simulink model "roll_control"  (R2020b)
settings: Solver=VariableStepAuto  StartTime=0.0  StopTime=3.45  FixedStep=0.001  RelTol=1e-5  AbsTol=1e-6
PostLoadFcn:
  | path = fileparts(which(bdroot))
  | cd(path)
  | masscgI = xlsread('mass,cg,I','mass,cg,I');
  | ThrustTable = xlsread('F15_Thrust','Sheet1');
  | u = xlsread('../../scp_new_problem/src/u.csv','u');
InitFcn:
  | HeightAboveSeaLevel = 5.4419142084;
  | 
  | GustStart = 1;
  | GustLength = [120, 130, 80];
  | GuestAmplitude = [ 2.5, -2.5,  1];
  | 
  | ShearSpeed = 4;
  | ShearDirection = 75;
  | 
  | Croll = 0.001 * (rand - 0.5);
  | Cyaw = 0.05 * (rand - 0.5);
  | Cside = 0.001 * (rand - 0.5);
  | 
  | GustStart = 2 * rand;
  | GustLength = [100 + 50 * (rand - 0.5), 100 + 50 * (rand - 0.5), 100 + 50 * (rand - 0.5)];
  | GuestAmplitude = [ 5 * (rand - 0.5), 5 * (rand - 0.5),  5 * (rand - 0.5)];
  | 
  | ShearSpeed = 5 * rand;
  | ShearDirection = 360 * rand;
  | 
  | HeightAboveSeaLevel = rand * 1000;
values from neighbouring files (symbols this model uses):
  cg = temp(4)    [NonlinearStateEstimationForActuatorDelay.m]
  D = zeros(size(B))    [RocketOutputFunction.m]    (also in StateSpaceController.m; TimeDelayCompensationElevator.m = [0; 0])
  F = eye(6)    [MEKFAttitudeOnly.m]
  I = reshape(x(1:9), [3 3])    [AdaptiveLQR.m]    (also in MEKF.m = diag([0.08 0.08 0.002]); MEKFAttitudeOnly.m = diag([0.08 0.08 0.002]); MEKF_old.m = diag([0.08 0.08 0.002]); NonlinearStateEstimationForActuatorDelay.m = diag([Ixx, Ixx, Izz]))
  K = 1.1    [DATCOMvsOR.m]    (also in Forces_and_Moments_Calculator.m; MEKF.m = (P * H.') / (H * P * H.' + V); MEKFAttitudeOnly.m = P2 * H' * inv(S); MEKF_old.m = (P * H.') / (H * P * H.' + V))
  mass = 1.0565    [ImpactVelocityNotParallelMatlab.m]    (also in NonlinearStateEstimationForActuatorDelay.m = temp(1); OneDLanding.m; RunImpactVelocityParforCompiled.m; StateSpaceController.m = 1.0616753546)
  q = x(13:16)    [AdaptiveLQR.m]    (also in MEKF.m = nominal_state(4:7); MEKFAttitudeOnly.m = [1 0 0 0]; MEKF_old.m = nominal_state(4:7); NonlinearStateEstimationForActuatorDelay.m = x(4:7))
  r = [0; 0; -(rocket_length - Average_cg)]    [StateSpaceController.m]    (also in TimeDelayCompensationElevator.m = [0;0]; Tracker.m)
  s = linspace(0, 100, nums)    [ImpactVelocityFunction.m]    (also in ImpactVelocityNotParallelMatlab.m = 1:5:500; ParallelImpactVelocity.m = .1:.01:500; ParralelRun.m = linspace(5,7, nums); RunImpactVelocityParforCompiled.m = 1:0.1:500)
  whentoignite = [s(row); v(col)]    [SecondPartLandingAlgorithm.m]
undefined symbols (not defined in the file or in its folder): Angle, Axis, deg, e0_0, e1_0, e2_0, e3_0, Earth, Kri, Light, magnitude, MIL, rad, WGS84
libraries: aerolibutil x7, vrlib x6, shared6dof x6, aerolibconvert2 x5, simulink x4, sharedtransform x4, aerolibwind2 x3, pid_lib x3, robotcorelib x2, sharedutil x2, aerolibasang x2, aerolibatmos2 x1
(part 1 of 3)
settings Model: ExtModeTrigDuration=100  OrderedModelArguments=off  Creator=rag  LastModifiedBy=rag
settings SolverCC: MaxConsecutiveZCs=10000  ZeroCrossAlgorithm=Adaptive  MinimalZcImpactIntegration=on
settings DataIOCC: Decimation=1000000  SaveOutput=off  DSMLogging=off  ReturnWorkspaceOutputs=off  StateSaveName=tmp_raccel_xout  SignalLoggingName=tmp_raccel_logsout  Refine=2
settings OptimizationCC: EfficientMapNaN2IntZero=off  SimCompilerOptimization=on
settings DebuggingCC: ReadBeforeWriteMsg=DisableAll  WriteAfterWriteMsg=DisableAll  WriteAfterReadMsg=DisableAll  AlgebraicLoopMsg=error
settings HardwareCC: ProdHWDeviceType=AMD->x86-64 (Windows64)  TargetBitPerPointer=64  TargetBitPerSizeT=64  TargetBitPerPtrDiffT=64  TargetLongLongMode=on  TargetIntDivRoundTo=Zero  TargetEndianess=LittleEndian  TargetWordSize=64  TargetHWDeviceType=MATLAB Host  ProdEqTarget=off
settings ModelReferenceCC: UpdateModelReferenceTargets=IfOutOfDate
settings SFSimCC: SFSimEcho=off  CustomCodeUndefinedFunction=UseInterfaceOnly
settings RTWCC: SystemTargetFile=raccel.tlc  TemplateMakefile=raccel_default_tmf  RTWVerbose=off  RTWUseSimCustomCode=on
settings CodeAppCC: GenerateComments=off  MaxIdLength=128  MangleLength=10
settings RaccelTargetCC: ENABLE_SLEXEC_SSBRIDGE=1  RTWCAPIParams=on  RTWCAPIRootIO=off
settings ConfigComp: CovScope=ReferencedModels

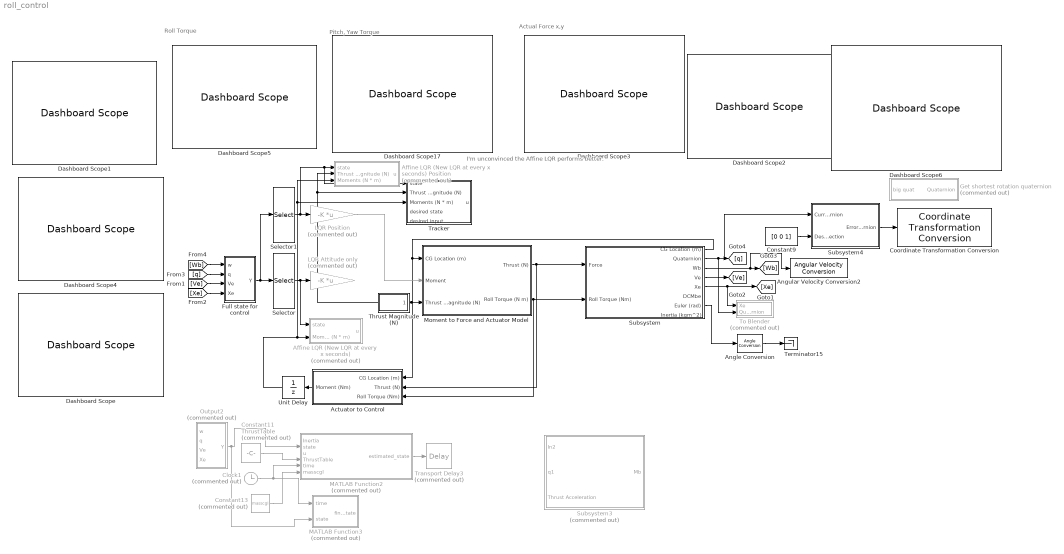
== system roll_control ==
  note: I'm unconvinced the Affine LQR performs better.
  note: Actual Force x,y
  note: Pitch, Yaw Torque
  note: Roll Torque
  Actuator to Control : Subsystem
  Affine LQR (New LQR at every x seconds) : Subsystem  Commented=on
  Affine LQR (New LQR at every x seconds) Position : Subsystem  Commented=on
  Angle Conversion : aerolibconvert2/Angle Conversion  IU=rad  OU=deg
  Angular Velocity Conversion2 : aerolibconvert2/Angular Velocity Conversion  IU=rad/s  OU=deg/s
  Clock1 : Clock  Commented=on
  Constant11 : Constant  Commented=on  Value=ThrustTable
  Constant13 : Constant  Commented=on  Value=masscgI
  Constant9 : Constant  Value=[0 0 1]
  Coordinate Transformation Conversion : robotcorelib/Coordinate Transformation Conversion  InputRepresentation=Quaternion  InputEulerSequence=ZYX  ShowTrVecInputPort=on  OutputRepresentation=Axis-Angle  OutputEulerSequence=ZYX  ShowTrVecOutputPort=on  SimulateUsing=Code generation
      settings: SourceProductBaseCode=NV,RO,RR,UV
  Dashboard Scope{,1..4,6} (6 alike) : DashboardScope
  Dashboard Scope17 : DashboardScope  TimeSpan=3.4500000000000002
  Dashboard Scope5 : DashboardScope  TimeSpan=3.4500000000000002
  Full state for control : Subsystem
  Get shortest rotation quaternion : Subsystem  Commented=on
  LQR Attitude only : Gain  Commented=on  Gain=-K  Multiplication=Matrix(K*u) (u vector)
  LQR Position : Gain  Commented=on  Gain=-K  Multiplication=Matrix(K*u) (u vector)
  MATLAB Function2 : MATLAB Function  Commented=on  TreatAsAtomicUnit=on
  MATLAB Function3 : MATLAB Function  Commented=on  TreatAsAtomicUnit=on
  Moment to Force and Actuator Model : Subsystem
  Output2 : Subsystem  Commented=on
  Selector : Selector  InputPortWidth=13  IndexOptions=Index vector (dialog)  Indices=[1:9]  OutputSizes=1
  Selector1 : Selector  InputPortWidth=13  IndexOptions=Index vector (dialog)  Indices=[1:6, 10:13]  OutputSizes=1
  Subsystem : Subsystem
  Subsystem3 : Subsystem  Commented=on
  Subsystem4 : Subsystem
  Terminator15 : Terminator
  Thrust Magnitude (N) : Subsystem
  To Blender : Subsystem  Commented=on
  Tracker : Subsystem
  Transport Delay3 : TransportDelay  Commented=on  DelayTime=0.5  TransDelayFeedthrough=on
  Unit Delay : UnitDelay  SampleTime=-1  HasFrameUpgradeWarning=on
  wires:
  Constant9/1 -> Subsystem4/2(Desired Direction)
  Constant11/1 -> MATLAB Function2/4(ThrustTable)
  Clock1/1 -> MATLAB Function2/5(time), MATLAB Function3/1(time)
  Output2/1(Y) -> MATLAB Function3/2(state), MATLAB Function2/2(state)
  Constant13/1 -> MATLAB Function2/6(masscgI)
  Subsystem/1(CG Location (m)) -> Actuator to Control/1(CG Location (m)), Moment to Force and Actuator Model/1(CG Location (m))
  Moment to Force and Actuator Model/1(Thrust (N)) -> Subsystem/1(Force), Actuator to Control/2(Thrust (N))
  Moment to Force and Actuator Model/2(Roll Torque (N m)) -> Subsystem/2(Roll Torque (Nm)), Actuator to Control/3(Roll Torque (Nm))
  MATLAB Function2/1(estimated_state) -> Transport Delay3/1
  Thrust Magnitude (N)/1(Thrust Magnitude (N)) -> Moment to Force and Actuator Model/3(Thrust Magnitude (N)), Affine LQR (New LQR at every x seconds) Position/2(Thrust Magnitude (N)), Tracker/2(Thrust Magnitude (N))
  Subsystem4/1(Error Quaternion) -> Coordinate Transformation Conversion/1
  Subsystem/5(Xe) -> To Blender/1(Xe), [Xe]
  [Xe] -> Full state for control/4(Xe)
  Subsystem/3(Wb) -> Angular Velocity Conversion2/1, [Wb]
  Subsystem/4(Ve) -> [Ve]
  Subsystem/2(Quaternion) -> To Blender/2(Quaternion), Subsystem4/1(Current Quaternion), [q]
  [Ve] -> Full state for control/3(Ve)
  [Wb] -> Full state for control/1(w)
  [q] -> Full state for control/2(q)
  Full state for control/1(Y) -> Selector1/1, Selector/1
  Selector/1 -> Affine LQR (New LQR at every x seconds)/1(state), LQR Attitude only/1
  Angle Conversion/1 -> Terminator15/1
  Subsystem/7(Euler (rad)) -> Angle Conversion/1
  Selector1/1 -> Tracker/1(state), Affine LQR (New LQR at every x seconds) Position/1(state), LQR Position/1
  Actuator to Control/1(Moment (Nm)) -> Unit Delay/1
  Unit Delay/1 -> Affine LQR (New LQR at every x seconds) Position/3(Moments (N * m)), Tracker/3(Moments (N * m)), Affine LQR (New LQR at every x seconds)/2(Moments (N * m))
  LQR Position/1 -> Moment to Force and Actuator Model/2(Moment)

== system roll_control/Actuator to Control ==
  CG Location (m) : Inport
  Thrust (N) : Inport  Port=2
  Roll Torque (Nm) : Inport  Port=3
  1 : Constant  Value=[0 0]
  Actuator to moment : Subsystem
  Mux : Mux  Inputs=2
  Sum : Sum  Inputs=|++
  Moment (Nm) : Outport
  wires:
  Actuator to moment/1(Thrust moment) -> Sum/1
  1/1 -> Mux/1
  Mux/1 -> Sum/2
  Roll Torque (Nm)/1 -> Mux/2
  Sum/1 -> Moment (Nm)/1
  CG Location (m)/1 -> Actuator to moment/1(CG Location (m))
  Thrust (N)/1 -> Actuator to moment/2(Thrust (N))

== system roll_control/Affine LQR (New LQR at every x seconds) ==
  state : Inport
  Moments (N * m) : Inport  Port=2
  Clock : Clock
  MATLAB Function1 : MATLAB Function  TreatAsAtomicUnit=on
  Matrix Multiply : Product  Multiplication=Matrix(*)
  Sum : Sum  Inputs=|--
  u : Outport
  wires:
  Clock/1 -> MATLAB Function1/3(time)
  state/1 -> Matrix Multiply/2, MATLAB Function1/1(state)
  Sum/1 -> u/1
  Matrix Multiply/1 -> Sum/1
  MATLAB Function1/2(k_0_out) -> Sum/2
  MATLAB Function1/1(K_x_out) -> Matrix Multiply/1
  Moments (N * m)/1 -> MATLAB Function1/2(u)

== system roll_control/Affine LQR (New LQR at every x seconds) Position ==
  state : Inport
  Thrust Magnitude (N) : Inport  Port=2
  Moments (N * m) : Inport  Port=3
  Clock : Clock
  MATLAB Function1 : MATLAB Function  TreatAsAtomicUnit=on
  Matrix Multiply : Product  Multiplication=Matrix(*)
  Sum : Sum  Inputs=|--
  u : Outport
  wires:
  Clock/1 -> MATLAB Function1/3(time)
  state/1 -> MATLAB Function1/1(state), Matrix Multiply/2
  Sum/1 -> u/1
  Matrix Multiply/1 -> Sum/1
  MATLAB Function1/2(k_0_out) -> Sum/2
  MATLAB Function1/1(K_x_out) -> Matrix Multiply/1
  Thrust Magnitude (N)/1 -> MATLAB Function1/4(Thrust_magnitude)
  Moments (N * m)/1 -> MATLAB Function1/2(u)

== system roll_control/Full state for control ==
  w : Inport
  q : Inport  Port=2
  Ve : Inport  Port=3
  Xe : Inport  Port=4
  Acos : Trigonometry  Commented=on  Operator=acos
  Derivative : Derivative  Commented=on
  Divide : Product  Commented=on  Inputs=**/
  Dot Product : DotProduct  Commented=on  SaturateOnIntegerOverflow=on  OutDataTypeStr=Inherit: Inherit via internal rule
  Gain : Gain  Commented=on  Gain=2
  Integrator : Integrator
  Selector : Selector  InputPortWidth=3  IndexOptions=Index vector (dialog)  Indices=[1 2]  OutputSizes=1
  Selector1 : Selector  InputPortWidth=4  IndexOptions=Index vector (dialog)  Indices=[2 3 4]  OutputSizes=1
  Selector2 : Selector  Commented=on  InputPortWidth=4  IndexOptions=Index vector (dialog)  Indices=1  OutputSizes=1
  Selector3 : Selector  InputPortWidth=3  IndexOptions=Index vector (dialog)  Indices=[1 2]  OutputSizes=1
  V : Math  Commented=on  Operator=sqrt  SignedPower=on  SaturateOnIntegerOverflow=on
  Vector Concatenate4 : Concatenate  NumInputs=5
  Y : Outport  VectorParamsAs1DForOutWhenUnconnected=off
  wires:
  Vector Concatenate4/1 -> Y/1
  Dot Product/1 -> V/1
  V/1 -> Divide/3
  Acos/1 -> Divide/1
  Selector2/1 -> Acos/1
  Divide/1 -> Derivative/1
  Derivative/1 -> Gain/1
  w/1 -> Vector Concatenate4/1
  q/1 -> Selector2/1, Selector1/1
  Selector1/1 -> Dot Product/2, Integrator/1, Vector Concatenate4/2, Dot Product/1
  Xe/1 -> Selector3/1
  Ve/1 -> Selector/1
  Selector/1 -> Vector Concatenate4/4
  Selector3/1 -> Vector Concatenate4/5
  Integrator/1 -> Vector Concatenate4/3

== system roll_control/Get shortest rotation quaternion ==
  big quat : Inport
  Gain : Gain  Gain=-1
  Selector3 : Selector  InputPortWidth=4  IndexOptions=Index vector (dialog)  Indices=1  OutputSizes=1
  Switch : Switch
  Quaternion : Outport  VectorParamsAs1DForOutWhenUnconnected=off
  wires:
  big quat/1 -> Switch/1, Gain/1, Selector3/1
  Switch/1 -> Quaternion/1
  Gain/1 -> Switch/3
  Selector3/1 -> Switch/2

== system roll_control/Moment to Force and Actuator Model ==
  note: 0.02 time delay and discretizing
  CG Location (m) : Inport
  Moment : Inport  Port=2
  Thrust Magnitude (N) : Inport  Port=3
  50Hz delay : MATLAB Function  Commented=on  TreatAsAtomicUnit=on
  Clock : Clock  Commented=on
      settings: Decimation=100
  "Delay, Discrete Servo" : Subsystem  Commented=on
  Moment to Force : Subsystem
  Saturation : Subsystem
  Thrust (N) : Outport
  Roll Torque (N m) : Outport  Port=2
  wires:
  CG Location (m)/1 -> Moment to Force/1(CG Location (m))
  Moment/1 -> Moment to Force/2(In2)
  Moment to Force/2(Roll Torque) -> Roll Torque (N m)/1
  Moment to Force/1(Desired Force x,y (N)) -> Saturation/1(Desired Force x,y (N))
  Thrust Magnitude (N)/1 -> Saturation/2(Thrust Magnitude (N))
  Saturation/1(Out1) -> Thrust (N)/1
  Clock/1 -> 50Hz delay/1(time)

== system roll_control/Output2 ==
  w : Inport
  " q" : Inport  Port=2
  Ve : Inport  Port=3
  Xe : Inport  Port=4
  Integrator1 : Integrator
  Selector1 : Selector  InputPortWidth=4  IndexOptions=Index vector (dialog)  Indices=[2 3 4]  OutputSizes=1
  Vector Concatenate4 : Concatenate  NumInputs=5
  Y : Outport  VectorParamsAs1DForOutWhenUnconnected=off
  wires:
  Vector Concatenate4/1 -> Y/1
  w/1 -> Vector Concatenate4/1
  " q"/1 -> Selector1/1, Vector Concatenate4/2
  Integrator1/1 -> Vector Concatenate4/3
  Selector1/1 -> Integrator1/1
  Xe/1 -> Vector Concatenate4/5
  Ve/1 -> Vector Concatenate4/4

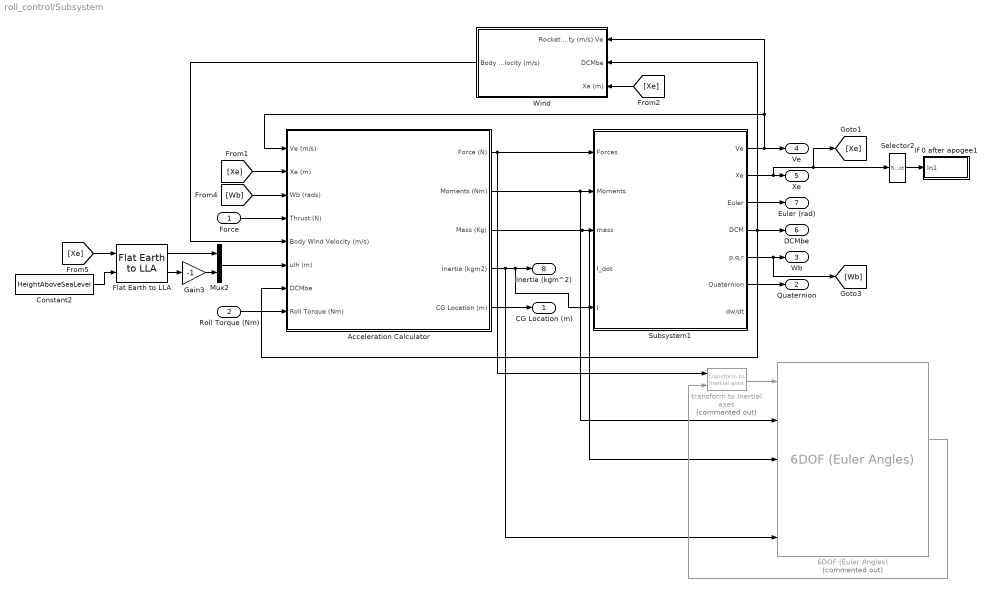
== system roll_control/Subsystem ==
  Force : Inport
  Roll Torque (Nm) : Inport  Port=2
  6DOF (Euler Angles) : shared6dof/6DOF (Euler Angles)  Commented=on  units=Metric (MKS)  mtype=Custom Variable  rep=Quaternion  xme_0=[0 0 0]  Vm_0=[0 0 0]  eul_0=[0 0 0]  pm_0=[0 0 0]  mass_0=1.0  mass_e=0.5  mass_f=2.0  inertia=eye(3)  inertia_e=eye(3)  inertia_f=2*eye(3)  k_quat=1.0  vre_flag=off  abi_flag=on  aMode=0  xme_statename=''  Vm_statename=''  eul_statename=''  quat_statename=''  pm_statename=''  mass_statename=''
      settings: SourceProductBaseCode=AE,PW,MT,UV,VE,VP
  Acceleration Calculator : Subsystem
  Constant2 : Constant  Value=HeightAboveSeaLevel
  Flat Earth to LLA : aerolibtransform2/Flat Earth to LLA  units=Metric (MKS)  ptype=Earth (WGS84)  F=1/298.257223563  R=6378137  refPosPort=off  LL0=[21.318358277648 -157.9232805920725]  psi=0
  Gain3 : Gain  Gain=-1
  If 0 after apogee1 : Subsystem
  Mux2 : Mux  Inputs=2
  Selector2 : Selector  InputPortWidth=3  IndexOptions=Index vector (dialog)  Indices=[3]  OutputSizes=1
  Subsystem1 : Subsystem
  Wind : Subsystem
  "transform to Inertial axes " : shared6dof/6DOF (Euler Angles)/transform to Inertial axes   Commented=on  SystemSampleTime=-1  VariantActivationTime=update diagram  Latency=0  AutoFrameSizeCalculation=off
      settings: SourceProductBaseCode=AE,PW,MT,UV,VE,VP
  CG Location (m) : Outport  VectorParamsAs1DForOutWhenUnconnected=off
  Quaternion : Outport  Port=2  VectorParamsAs1DForOutWhenUnconnected=off
  Wb : Outport  Port=3  VectorParamsAs1DForOutWhenUnconnected=off
  Ve : Outport  Port=4  VectorParamsAs1DForOutWhenUnconnected=off
  Xe : Outport  Port=5  VectorParamsAs1DForOutWhenUnconnected=off
  DCMbe : Outport  Port=6  VectorParamsAs1DForOutWhenUnconnected=off
  Euler (rad) : Outport  Port=7  VectorParamsAs1DForOutWhenUnconnected=off
  Inertia (kgm^2) : Outport  Port=8  VectorParamsAs1DForOutWhenUnconnected=off
  wires:
  Flat Earth to LLA/1 -> Mux2/1
  Flat Earth to LLA/2 -> Gain3/1
  Gain3/1 -> Mux2/2
  Mux2/1 -> Acceleration Calculator/6(ulh (m))
  Constant2/1 -> Flat Earth to LLA/2
  [Xe] -> Acceleration Calculator/2(Xe (m))
  Selector2/1 -> If 0 after apogee1/1(In1)
  [Xe] -> Flat Earth to LLA/1
  [Wb] -> Acceleration Calculator/3(Wb (rads))
  Acceleration Calculator/5(CG Location (m)) -> CG Location (m)/1
  Acceleration Calculator/4(Inertia (kgm2)) -> 6DOF (Euler Angles)/5, Subsystem1/5(I), Inertia (kgm^2)/1
  Acceleration Calculator/1(Force (N)) -> Subsystem1/1(Forces), "transform to Inertial axes "/1
  Roll Torque (Nm)/1 -> Acceleration Calculator/8(Roll Torque (Nm))
  Subsystem1/1(Ve) -> Acceleration Calculator/1(Ve (m/s)), Wind/1(Rocket velocity (m/s) Ve), Ve/1
  Subsystem1/5(p,q,r) -> [Wb], Wb/1
  Subsystem1/3(Euler) -> Euler (rad)/1
  Wind/1(Body Wind Velocity (m/s)) -> Acceleration Calculator/5(Body Wind Velocity (m/s))
  Subsystem1/6(Quaternion) -> Quaternion/1
  Subsystem1/4(DCM) -> Wind/2(DCMbe), Acceleration Calculator/7(DCMbe), DCMbe/1
  Acceleration Calculator/2(Moments (Nm)) -> 6DOF (Euler Angles)/2, Subsystem1/2(Moments)
  Force/1 -> Acceleration Calculator/4(Thrust (N))
  Subsystem1/2(Xe) -> [Xe], Selector2/1, Xe/1
  [Xe] -> Wind/3(Xe (m))
  Acceleration Calculator/3(Mass (Kg)) -> 6DOF (Euler Angles)/3, Subsystem1/3(mass)
  "transform to Inertial axes "/1 -> 6DOF (Euler Angles)/1
  6DOF (Euler Angles)/4 -> "transform to Inertial axes "/2

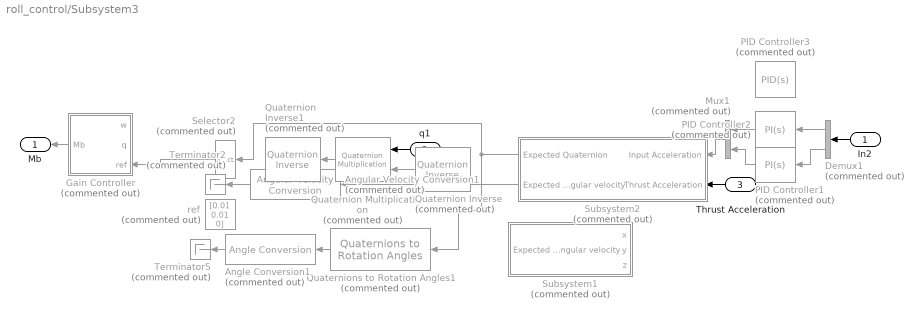
== system roll_control/Subsystem3 ==
  In2 : Inport
  q1 : Inport  Port=2
  Thrust Acceleration : Inport  Port=3
  Angle Conversion1 : aerolibconvert2/Angle Conversion  Commented=on  IU=rad  OU=deg
  Angular Velocity Conversion1 : aerolibconvert2/Angular Velocity Conversion  Commented=on  IU=rad/s  OU=deg/s
  Demux1 : Demux  Commented=on  Outputs=2
  Gain Controller : Subsystem  Commented=on
  Mux1 : Mux  Commented=on  Inputs=2
  PID Controller1 : pid_lib/PID Controller  Commented=on  Controller=PI  Form=Parallel  TimeDomain=Continuous-time  UseExternalTs=off  SampleTime=-1  IntegratorMethod=Forward Euler  FilterMethod=Forward Euler  ControllerParametersSource=internal  P=-.75  I=-.3  D=0  UseFilter=on  N=10000  TunerSelectOption=Transfer Function Based (PID Tuner App)  InitialConditionSource=internal  InitialConditionForIntegrator=0  InitialConditionForFilter=0  DifferentiatorICPrevScaledInput=0  ExternalReset=none  TrackingMode=off  Kt=1  LimitOutput=off  SatLimitsSource=internal  UpperSaturationLimit=inf  LowerSaturationLimit=-inf  LinearizeAsGain=on  AntiWindupMode=none  Kb=1  POutMin=[]  POutMax=[]  IOutMin=[]  IOutMax=[]  DOutMin=[]  DOutMax=[]  NOutMin=[]  NOutMax=[]  SumOutMin=[]  SumOutMax=[]  SaturationOutMin=[]  SaturationOutMax=[]  PParamMin=[]  PParamMax=[]  IParamMin=[]  IParamMax=[]  DParamMin=[]  DParamMax=[]  NParamMin=[]  NParamMax=[]  KbParamMin=[]  KbParamMax=[]  KtParamMin=[]  KtParamMax=[]  KbOutMin=[]  KbOutMax=[]  KtOutMin=[]  KtOutMax=[]  IntegratorOutMin=[]  IntegratorOutMax=[]  FilterOutMin=[]  FilterOutMax=[]  SumI1OutMin=[]  SumI1OutMax=[]  SumI2OutMin=[]  SumI2OutMax=[]  SumI3OutMin=[]  SumI3OutMax=[]  SumI4OutMin=[]  SumI4OutMax=[]  SumDOutMin=[]  SumDOutMax=[]  DifferentiatorOutMin=[]  DifferentiatorOutMax=[]  FilterDiffOutCoefMin=[]  FilterDiffOutCoefMax=[]  ReciprocalOutMin=[]  ReciprocalOutMax=[]  SumDenOutMin=[]  SumDenOutMax=[]  SumNumOutMin=[]  SumNumOutMax=[]  DivideOutMin=[]  DivideOutMax=[]  UdiffTsProdOutMin=[]  UdiffTsProdOutMax=[]  NTsProdOutMin=[]  NTsProdOutMax=[]  UintegralTsProdOutMin=[]  UintegralTsProdOutMax=[]  UngainTsProdOutMin=[]  UngainTsProdOutMax=[]  IntegratorContinuousStateAttributes=''  IntegratorStateMustResolveToSignalObject=off  IntegratorRTWStateStorageClass=Auto  FilterContinuousStateAttributes=''  FilterStateMustResolveToSignalObject=off  FilterRTWStateStorageClass=Auto  ParallelPVariant=InternalParameters  IdealPVariant=Disabled  IVariant=InternalParameters  DVariant=Disabled  IntegratorVariant=Continuous  SatVariant=Disabled  AWVariant=Passthrough  PCopyVariant=Disabled  TRVariant=Disabled  FdbkBlocksVariant=Forward  IdealPFdbkVariant=Disabled  SatFdbkVariant=Disabled  DerivativeFilterVariant=Disabled  NVariant=Disabled  NCopyVariant=Disabled_SignalSpec  FilterICVariant=Disabled  IntegratorICVariant=InternalICs  ExternalResetVariant=Disabled  TRSumVariant=Passthrough  SumFdbkVariant=Disabled  SumVariant=Sum_PI  TsampFilterVariant=InternalTs  TsampNgainVariant=Passthrough  TsampIntegralVariant=Passthrough  ExternalSaturationOutDataTypeStr=Inherit: Same as second input
  PID Controller2 : pid_lib/PID Controller  Commented=on  Controller=PI  Form=Parallel  TimeDomain=Continuous-time  UseExternalTs=off  SampleTime=-1  IntegratorMethod=Forward Euler  FilterMethod=Forward Euler  ControllerParametersSource=internal  P=-.75  I=-.3  D=0  UseFilter=on  N=10000  TunerSelectOption=Transfer Function Based (PID Tuner App)  InitialConditionSource=internal  InitialConditionForIntegrator=0  InitialConditionForFilter=0  DifferentiatorICPrevScaledInput=0  ExternalReset=none  TrackingMode=off  Kt=1  LimitOutput=off  SatLimitsSource=internal  UpperSaturationLimit=inf  LowerSaturationLimit=-inf  LinearizeAsGain=on  AntiWindupMode=none  Kb=1  POutMin=[]  POutMax=[]  IOutMin=[]  IOutMax=[]  DOutMin=[]  DOutMax=[]  NOutMin=[]  NOutMax=[]  SumOutMin=[]  SumOutMax=[]  SaturationOutMin=[]  SaturationOutMax=[]  PParamMin=[]  PParamMax=[]  IParamMin=[]  IParamMax=[]  DParamMin=[]  DParamMax=[]  NParamMin=[]  NParamMax=[]  KbParamMin=[]  KbParamMax=[]  KtParamMin=[]  KtParamMax=[]  KbOutMin=[]  KbOutMax=[]  KtOutMin=[]  KtOutMax=[]  IntegratorOutMin=[]  IntegratorOutMax=[]  FilterOutMin=[]  FilterOutMax=[]  SumI1OutMin=[]  SumI1OutMax=[]  SumI2OutMin=[]  SumI2OutMax=[]  SumI3OutMin=[]  SumI3OutMax=[]  SumI4OutMin=[]  SumI4OutMax=[]  SumDOutMin=[]  SumDOutMax=[]  DifferentiatorOutMin=[]  DifferentiatorOutMax=[]  FilterDiffOutCoefMin=[]  FilterDiffOutCoefMax=[]  ReciprocalOutMin=[]  ReciprocalOutMax=[]  SumDenOutMin=[]  SumDenOutMax=[]  SumNumOutMin=[]  SumNumOutMax=[]  DivideOutMin=[]  DivideOutMax=[]  UdiffTsProdOutMin=[]  UdiffTsProdOutMax=[]  NTsProdOutMin=[]  NTsProdOutMax=[]  UintegralTsProdOutMin=[]  UintegralTsProdOutMax=[]  UngainTsProdOutMin=[]  UngainTsProdOutMax=[]  IntegratorContinuousStateAttributes=''  IntegratorStateMustResolveToSignalObject=off  IntegratorRTWStateStorageClass=Auto  FilterContinuousStateAttributes=''  FilterStateMustResolveToSignalObject=off  FilterRTWStateStorageClass=Auto  ParallelPVariant=InternalParameters  IdealPVariant=Disabled  IVariant=InternalParameters  DVariant=Disabled  IntegratorVariant=Continuous  SatVariant=Disabled  AWVariant=Passthrough  PCopyVariant=Disabled  TRVariant=Disabled  FdbkBlocksVariant=Forward  IdealPFdbkVariant=Disabled  SatFdbkVariant=Disabled  DerivativeFilterVariant=Disabled  NVariant=Disabled  NCopyVariant=Disabled_SignalSpec  FilterICVariant=Disabled  IntegratorICVariant=InternalICs  ExternalResetVariant=Disabled  TRSumVariant=Passthrough  SumFdbkVariant=Disabled  SumVariant=Sum_PI  TsampFilterVariant=InternalTs  TsampNgainVariant=Passthrough  TsampIntegralVariant=Passthrough  ExternalSaturationOutDataTypeStr=Inherit: Same as second input
  PID Controller3 : pid_lib/PID Controller  Commented=on  Controller=PID  Form=Parallel  TimeDomain=Continuous-time  UseExternalTs=off  SampleTime=-1  IntegratorMethod=Forward Euler  FilterMethod=Forward Euler  ControllerParametersSource=internal  P=-0.123834085166626  I=-0.0589771468563032  D=0.0137648749687481  UseFilter=on  N=8.99638285475018  TunerSelectOption=Transfer Function Based (PID Tuner App)  InitialConditionSource=internal  InitialConditionForIntegrator=0  InitialConditionForFilter=0  DifferentiatorICPrevScaledInput=0  ExternalReset=none  TrackingMode=off  Kt=1  LimitOutput=off  SatLimitsSource=internal  UpperSaturationLimit=inf  LowerSaturationLimit=-inf  LinearizeAsGain=on  AntiWindupMode=none  Kb=1  POutMin=[]  POutMax=[]  IOutMin=[]  IOutMax=[]  DOutMin=[]  DOutMax=[]  NOutMin=[]  NOutMax=[]  SumOutMin=[]  SumOutMax=[]  SaturationOutMin=[]  SaturationOutMax=[]  PParamMin=[]  PParamMax=[]  IParamMin=[]  IParamMax=[]  DParamMin=[]  DParamMax=[]  NParamMin=[]  NParamMax=[]  KbParamMin=[]  KbParamMax=[]  KtParamMin=[]  KtParamMax=[]  KbOutMin=[]  KbOutMax=[]  KtOutMin=[]  KtOutMax=[]  IntegratorOutMin=[]  IntegratorOutMax=[]  FilterOutMin=[]  FilterOutMax=[]  SumI1OutMin=[]  SumI1OutMax=[]  SumI2OutMin=[]  SumI2OutMax=[]  SumI3OutMin=[]  SumI3OutMax=[]  SumI4OutMin=[]  SumI4OutMax=[]  SumDOutMin=[]  SumDOutMax=[]  DifferentiatorOutMin=[]  DifferentiatorOutMax=[]  FilterDiffOutCoefMin=[]  FilterDiffOutCoefMax=[]  ReciprocalOutMin=[]  ReciprocalOutMax=[]  SumDenOutMin=[]  SumDenOutMax=[]  SumNumOutMin=[]  SumNumOutMax=[]  DivideOutMin=[]  DivideOutMax=[]  UdiffTsProdOutMin=[]  UdiffTsProdOutMax=[]  NTsProdOutMin=[]  NTsProdOutMax=[]  UintegralTsProdOutMin=[]  UintegralTsProdOutMax=[]  UngainTsProdOutMin=[]  UngainTsProdOutMax=[]  IntegratorContinuousStateAttributes=''  IntegratorStateMustResolveToSignalObject=off  IntegratorRTWStateStorageClass=Auto  FilterContinuousStateAttributes=''  FilterStateMustResolveToSignalObject=off  FilterRTWStateStorageClass=Auto  ParallelPVariant=InternalParameters  IdealPVariant=Disabled  IVariant=InternalParameters  DVariant=InternalParameters  IntegratorVariant=Continuous  SatVariant=Disabled  AWVariant=Passthrough  PCopyVariant=Disabled  TRVariant=Disabled  FdbkBlocksVariant=Forward  IdealPFdbkVariant=Disabled  SatFdbkVariant=Disabled  DerivativeFilterVariant=ContFilter  NVariant=InternalParameters  NCopyVariant=Disabled  FilterICVariant=InternalICsFilter  IntegratorICVariant=InternalICs  ExternalResetVariant=Disabled  TRSumVariant=Passthrough  SumFdbkVariant=Disabled  SumVariant=Sum_PID  TsampFilterVariant=InternalTs  TsampNgainVariant=Passthrough  TsampIntegralVariant=Passthrough  ExternalSaturationOutDataTypeStr=Inherit: Same as second input
  Quaternion Inverse : aerolibutil/Quaternion Inverse  Commented=on
  Quaternion Inverse1 : aerolibutil/Quaternion Inverse  Commented=on
  Quaternion Multiplication : aerolibutil/Quaternion Multiplication  Commented=on
  Quaternions to Rotation Angles1 : sharedtransform/Quaternions to Rotation Angles  Commented=on  rotationOrder=XYZ  aMode=aMode
      settings: SourceProductBaseCode=AE,PW,MT,UV,VE,VP
  Selector2 : Selector  Commented=on  InputPortWidth=4  IndexOptions=Index vector (dialog)  Indices=[3 2 4]  OutputSizes=1
  Subsystem1 : Subsystem  Commented=on
  Subsystem2 : Subsystem  Commented=on
  Terminator2 : Terminator  Commented=on
  Terminator5 : Terminator  Commented=on
  ref : Constant  Commented=on  Value=[0.01 0.01 0]
  Mb : Outport
  wires:
  Quaternion Inverse/1 -> Quaternion Multiplication/2
  Subsystem2/2(Expected angular velocity) -> Angular Velocity Conversion1/1
  Quaternion Multiplication/1 -> Quaternion Inverse1/1
  Selector2/1 -> Gain Controller/3(ref)
  Angular Velocity Conversion1/1 -> Terminator2/1
  Quaternions to Rotation Angles1/1 -> Angle Conversion1/1
  Demux1/2 -> PID Controller1/1
  PID Controller2/1 -> Mux1/1
  Mux1/1 -> Subsystem2/1(Input Acceleration)
  Subsystem2/1(Expected Quaternion) -> Selector2/1, Quaternions to Rotation Angles1/1
  PID Controller1/1 -> Mux1/2
  Angle Conversion1/1 -> Terminator5/1
  Demux1/1 -> PID Controller2/1
  In2/1 -> Demux1/1
  q1/1 -> Quaternion Multiplication/1
  Gain Controller/1(Mb) -> Mb/1
  Thrust Acceleration/1 -> Subsystem2/2(Thrust Acceleration)

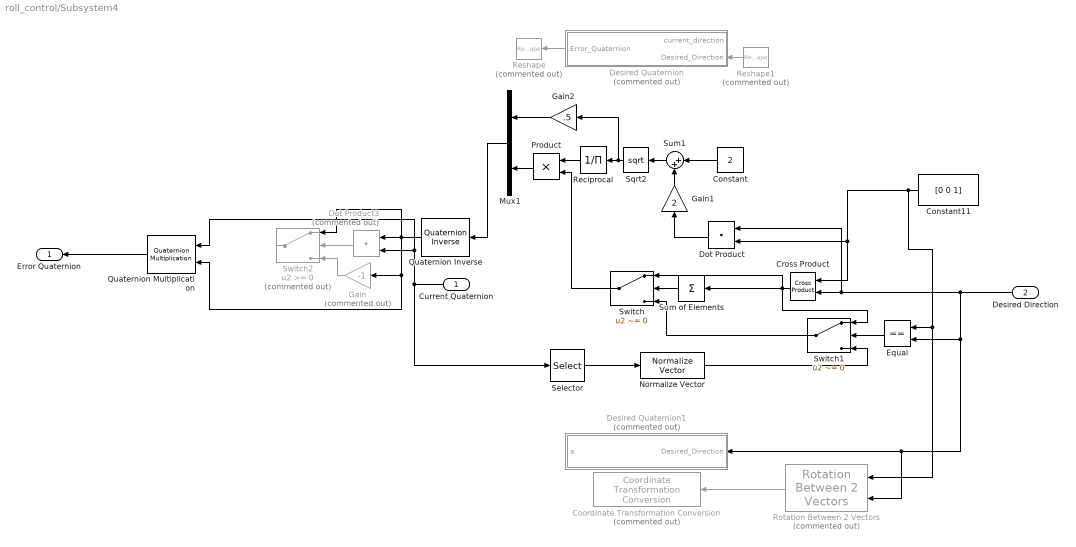
== system roll_control/Subsystem4 ==
  Current Quaternion : Inport
  Desired Direction : Inport  Port=2
  Constant : Constant  Value=2
  Constant11 : Constant  Value=[0 0 1]
  Coordinate Transformation Conversion : robotcorelib/Coordinate Transformation Conversion  Commented=on  InputRepresentation=Axis-Angle  InputEulerSequence=ZYX  ShowTrVecInputPort=on  OutputRepresentation=Quaternion  OutputEulerSequence=ZYX  ShowTrVecOutputPort=on  SimulateUsing=Code generation
      settings: SourceProductBaseCode=NV,RO,RR,UV
  Cross Product : vrlib/Utilities/Cross Product
  Desired Quaternion : MATLAB Function  Commented=on  TreatAsAtomicUnit=on
  Desired Quaternion1 : MATLAB Function  Commented=on  TreatAsAtomicUnit=on
  Dot Product : DotProduct  InputSameDT=on  OutDataTypeStr=Inherit: Inherit via internal rule
  Dot Product3 : DotProduct  Commented=on  InputSameDT=on  OutDataTypeStr=Inherit: Inherit via internal rule
  Equal : RelationalOperator  Operator===  OutDataTypeStr=boolean  RndMeth=Simplest
  Gain : Gain  Commented=on  Gain=-1
  Gain1 : Gain  Gain=2
  Gain2 : Gain  Gain=.5
  Mux1 : Mux  Inputs=2
  Normalize Vector : vrlib/Utilities/Normalize Vector  maxzero=0
  Product : Product
  Quaternion Inverse : aerolibutil/Quaternion Inverse
  Quaternion Multiplication : aerolibutil/Quaternion Multiplication
  Reciprocal : Product  Inputs=/
  Reshape : Reshape  Commented=on
  Reshape1 : Reshape  Commented=on  OutputDimensionality=Row vector (2-D)
  Rotation Between 2 Vectors : vrlib/Utilities/Rotation Between 2 Vectors  Commented=on
      settings: SourceProductBaseCode=SL
  Selector : Selector  InputPortWidth=4  IndexOptions=Index vector (dialog)  Indices="[2  3 4]"  OutputSizes=1
  Sqrt2 : Sqrt  SaturateOnIntegerOverflow=on
  Sum of Elements : Sum  Inputs=+
  Sum1 : Sum  Inputs=|++
  Switch : Switch  Criteria=u2 ~= 0
  Switch1 : Switch  Criteria=u2 ~= 0
  Switch2 : Switch  Commented=on
  Error Quaternion : Outport  VectorParamsAs1DForOutWhenUnconnected=off
  wires:
  Reshape1/1 -> Desired Quaternion/2(Desired_Direction)
  Constant11/1 -> Cross Product/1, Dot Product/2, Equal/1, Rotation Between 2 Vectors/1
  Desired Quaternion/1(Error_Quaternion) -> Reshape/1
  Desired Direction/1 -> Dot Product/1, Cross Product/2, Rotation Between 2 Vectors/2, Desired Quaternion1/1(Desired_Direction), Equal/2
  Cross Product/1 -> Switch/1, Sum of Elements/1, Switch1/1
  Dot Product/1 -> Gain1/1
  Current Quaternion/1 -> Selector/1, Quaternion Multiplication/1, Dot Product3/2
  Selector/1 -> Normalize Vector/1
  Equal/1 -> Switch1/2
  Switch1/1 -> Switch/3
  Quaternion Inverse/1 -> Quaternion Multiplication/2, Gain/1, Switch2/1, Dot Product3/1
  Dot Product3/1 -> Switch2/2
  Gain/1 -> Switch2/3
  Quaternion Multiplication/1 -> Error Quaternion/1
  Sum1/1 -> Sqrt2/1
  Gain1/1 -> Sum1/2
  Constant/1 -> Sum1/1
  Sqrt2/1 -> Gain2/1, Reciprocal/1
  Reciprocal/1 -> Product/1
  Product/1 -> Mux1/2
  Gain2/1 -> Mux1/1
  Normalize Vector/1 -> Switch1/3
  Rotation Between 2 Vectors/1 -> Coordinate Transformation Conversion/1
  Mux1/1 -> Quaternion Inverse/1
  Sum of Elements/1 -> Switch/2
  Switch/1 -> Product/2

== system roll_control/Thrust Magnitude (N) ==
  Clock : Clock
      settings: Decimation=100
  Constant : Constant
  Constant5 : Constant  Commented=on  Value=whentoignite
  Constant8 : Constant  Commented=on  Value=3.45
  GreaterThan1 : RelationalOperator  Commented=on  Operator=>  OutDataTypeStr=boolean  RndMeth=Simplest
  Integrator : Integrator  Commented=on
  MATLAB Function : MATLAB Function  Commented=on  TreatAsAtomicUnit=on
  Product : Product
  Switch : Switch  Criteria=u2 > Threshold  Threshold=3.45
  Thrust : Lookup_n-D  NumberOfTableDimensions=1  BreakpointsForDimension1=ThrustTable(:,1)  BreakpointsForDimension1FirstPoint=0  BreakpointsForDimension1Spacing=1.5e-5  Table=ThrustTable(:,2)  ExtrapMethod=Clip  InternalRulePriority=Speed  RndMeth=Simplest  InputSameDT=on
  Thrust1 : Lookup_n-D  Commented=on  NumberOfTableDimensions=1  BreakpointsForDimension1=ThrustTable(:,1)  BreakpointsForDimension1FirstPoint=0  BreakpointsForDimension1Spacing=1.5e-5  Table=ThrustTable(:,2)  ExtrapMethod=Clip  InternalRulePriority=Speed  RndMeth=Simplest  InputSameDT=on
  White Noise : RandomNumber  Commented=on  DisableCoverage=on  Mean=1  Variance=0.001  Seed=21359  SampleTime=0.01
  Thrust Magnitude (N) : Outport
  wires:
  GreaterThan1/1 -> MATLAB Function/2(incoastingphase)
  Clock/1 -> GreaterThan1/1, Switch/2, Thrust/1
  Constant/1 -> Product/2
  Thrust/1 -> Product/1
  Switch/1 -> Thrust Magnitude (N)/1
  Integrator/1 -> Thrust1/1
  MATLAB Function/1(y) -> Integrator/1
  Constant8/1 -> GreaterThan1/2
  Constant5/1 -> MATLAB Function/1(whentoignite)
  Product/1 -> Switch/3

== system roll_control/To Blender ==
  Xe : Inport
  Quaternion : Inport  Port=2
  Mux : Mux  Inputs=2
  To File : ToFile  Filename=Blender  MatrixName=data  SaveFormat=Timeseries
  wires:
  Xe/1 -> Mux/1
  Quaternion/1 -> Mux/2
  Mux/1 -> To File/1

== system roll_control/Tracker ==
  state : Inport
  Thrust Magnitude (N) : Inport  Port=2
  Moments (N * m) : Inport  Port=3
  desired state : Inport  Port=4
  desired input : Inport  Port=5
  Clock : Clock
  MATLAB Function1 : MATLAB Function  TreatAsAtomicUnit=on
  Matrix Multiply : Product  Multiplication=Matrix(*)
  Sum : Sum  Inputs=|--
  u : Outport
  wires:
  Clock/1 -> MATLAB Function1/3(time)
  state/1 -> Matrix Multiply/2, MATLAB Function1/1(state)
  Sum/1 -> u/1
  Matrix Multiply/1 -> Sum/1
  MATLAB Function1/2(k_0_out) -> Sum/2
  MATLAB Function1/1(K_x_out) -> Matrix Multiply/1
  Thrust Magnitude (N)/1 -> MATLAB Function1/4(Thrust_magnitude)
  Moments (N * m)/1 -> MATLAB Function1/2(u)
  desired input/1 -> MATLAB Function1/6(u_d)
  desired state/1 -> MATLAB Function1/5(x_d)

== system roll_control/Actuator to Control/Actuator to moment ==
  CG Location (m) : Inport
  Thrust (N) : Inport  Port=2
  1 : Constant  Value=[0 0]
  Constant3 : Constant  Value=.95
  Cross Product : vrlib/Utilities/Cross Product
  Gain : Gain  Gain=-1
  Mux : Mux  Inputs=2
  Sum1 : Sum  Inputs=-+|
  Thrust moment : Outport  VectorParamsAs1DForOutWhenUnconnected=off
  wires:
  Constant3/1 -> Sum1/2
  CG Location (m)/1 -> Sum1/1
  Mux/1 -> Cross Product/1
  Sum1/1 -> Gain/1
  1/1 -> Mux/1
  Thrust (N)/1 -> Cross Product/2
  Cross Product/1 -> Thrust moment/1
  Gain/1 -> Mux/2

== system roll_control/Moment to Force and Actuator Model/Delay, Discrete Servo ==
  In1 : Inport
  In3 : Inport  Port=2
  Rate Transition : RateTransition  OutPortSampleTime=0.02
  Transport Delay : TransportDelay  DelayTime=0.07  TransDelayFeedthrough=on
  Transport Delay1 : TransportDelay  DelayTime=0.01  TransDelayFeedthrough=on
  Out3 : Outport
  Output : Outport  Port=2
  wires:
  Rate Transition/1 -> Transport Delay/1
  Transport Delay/1 -> Output/1
  In1/1 -> Rate Transition/1
  Transport Delay1/1 -> Out3/1
  In3/1 -> Transport Delay1/1

== system roll_control/Moment to Force and Actuator Model/Moment to Force ==
  CG Location (m) : Inport
  In2 : Inport  Port=2
  Constant14 : Constant  Value=[0 1; -1 0]
  Constant3 : Constant  Value=.95
  Demux2 : Demux  Outputs=3
  Force : Product  Multiplication=Matrix(*)
  Gain : Gain  Gain=-1
  Moment to Force : Product  Inputs=/*
  Mux2 : Mux  Inputs=2
  Sum1 : Sum  Inputs=-+|
  Desired Force x,y (N) : Outport
  Roll Torque : Outport  Port=2
  wires:
  Demux2/2 -> Mux2/2
  Mux2/1 -> Moment to Force/2
  Constant3/1 -> Sum1/2
  Moment to Force/1 -> Force/2
  Demux2/3 -> Roll Torque/1
  Constant14/1 -> Force/1
  Demux2/1 -> Mux2/1
  Sum1/1 -> Gain/1
  CG Location (m)/1 -> Sum1/1
  In2/1 -> Demux2/1
  Force/1 -> Desired Force x,y (N)/1
  Gain/1 -> Moment to Force/1

== system roll_control/Moment to Force and Actuator Model/Saturation ==
  note: Thrust x,y component
  note: Thrust z component
  Desired Force x,y (N) : Inport
  Thrust Magnitude (N) : Inport  Port=2
  Dot Product : DotProduct  SaturateOnIntegerOverflow=on  OutDataTypeStr=Inherit: Inherit via internal rule
  Dot Product1 : DotProduct  SaturateOnIntegerOverflow=on  OutDataTypeStr=Inherit: Inherit via internal rule
  Gain : Gain  Gain=sin(deg2rad(5))
  If 0 after apogee2 : Subsystem  Commented=on
  MinMax1 : MinMax  Inputs=2
  Multiply1 : Product  Inputs=**
  Mux : Mux  Inputs=2
  Normalize Vector : vrlib/Utilities/Normalize Vector  maxzero=0
  Square : Math  Operator=square  SignedPower=on  SaturateOnIntegerOverflow=on
  Subtract : Sum  Inputs=-+
  V : Math  Operator=sqrt  SignedPower=on  SaturateOnIntegerOverflow=on
  V1 : Math  Operator=sqrt  SignedPower=on  SaturateOnIntegerOverflow=on
  Out1 : Outport
  wires:
  V/1 -> Mux/2
  Gain/1 -> MinMax1/2
  Desired Force x,y (N)/1 -> Normalize Vector/1, Dot Product1/1, Dot Product1/2
  Dot Product/1 -> Subtract/1
  Square/1 -> Subtract/2
  Subtract/1 -> V/1
  Multiply1/1 -> Mux/1, Dot Product/2, Dot Product/1
  Dot Product1/1 -> V1/1
  V1/1 -> MinMax1/1
  MinMax1/1 -> Multiply1/2
  Normalize Vector/1 -> Multiply1/1
  Thrust Magnitude (N)/1 -> Square/1, Gain/1
  Mux/1 -> Out1/1

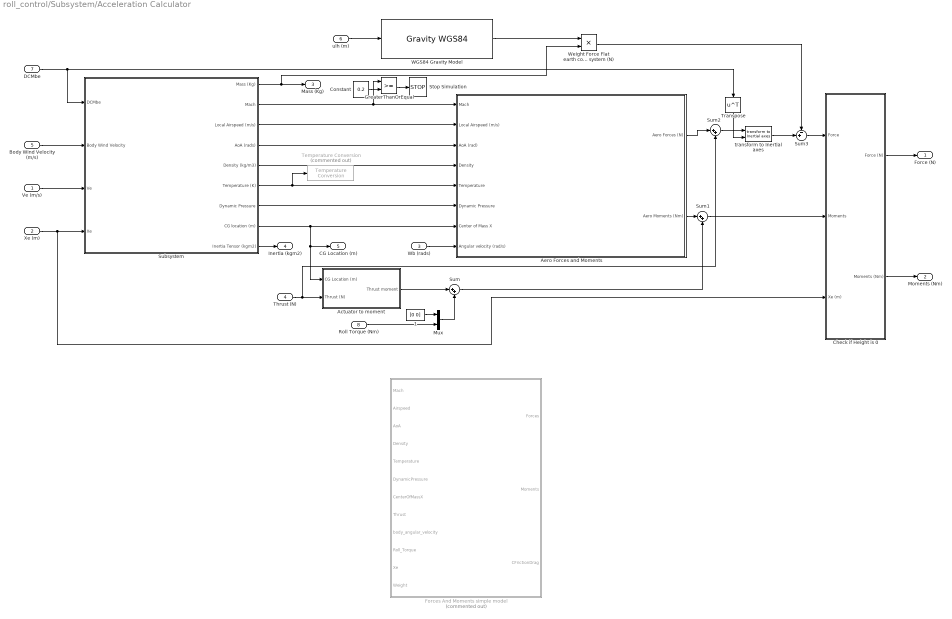
== system roll_control/Subsystem/Acceleration Calculator ==
  Ve (m/s) : Inport
  Xe (m) : Inport  Port=2
  Wb (rads) : Inport  Port=3
  Thrust (N) : Inport  Port=4
  Body Wind Velocity (m/s) : Inport  Port=5
  ulh (m) : Inport  Port=6  PortDimensions=3
  DCMbe : Inport  Port=7
  Roll Torque (Nm) : Inport  Port=8
  1 : Constant  Value=[0 0]
  Actuator to moment : Subsystem
  Aero Forces and Moments : Subsystem
  Check if Height is 0 : Subsystem
  Constant : Constant  Value=0.2
  Forces And Moments simple model : MATLAB Function  Commented=on  TreatAsAtomicUnit=on
  GreaterThanOrEqual : RelationalOperator  OutDataTypeStr=boolean  RndMeth=Simplest
  Mux : Mux  Inputs=2
  Stop Simulation : Stop
  Subsystem : Subsystem
  Sum : Sum  Inputs=|++
  Sum1 : Sum  Inputs=|++
  Sum2 : Sum  Inputs=|++
  Sum3 : Sum  Inputs=-+|
  Temperature Conversion : aerolibconvert2/Temperature Conversion  Commented=on  IU=K  OU=C
      settings: SourceProductBaseCode=AE
  Transpose : Math  Operator=transpose  SignedPower=on  SaturateOnIntegerOverflow=on
  "WGS84 Gravity Model  " : GravityWGS84
  Weight Force Flat earth coordinate system (N) : Product
  "transform to Inertial axes " : shared6dof/6DOF (Euler Angles)/transform to Inertial axes   SystemSampleTime=-1  VariantActivationTime=update diagram  Latency=0  AutoFrameSizeCalculation=off
      settings: SourceProductBaseCode=AE,PW,MT,UV,VE,VP
  Force (N) : Outport  VectorParamsAs1DForOutWhenUnconnected=off
  Moments (Nm) : Outport  Port=2  VectorParamsAs1DForOutWhenUnconnected=off
  Mass (Kg) : Outport  Port=3  VectorParamsAs1DForOutWhenUnconnected=off
  Inertia (kgm2) : Outport  Port=4  VectorParamsAs1DForOutWhenUnconnected=off
  CG Location (m) : Outport  Port=5  VectorParamsAs1DForOutWhenUnconnected=off
  wires:
  Ve (m/s)/1 -> Subsystem/3(Ve)
  Subsystem/9(Inertia Tensor (kgm2)) -> Inertia (kgm2)/1
  Subsystem/1(Mass (Kg)) -> Weight Force Flat earth coordinate system (N)/2, Mass (Kg)/1
  DCMbe/1 -> Transpose/1, Subsystem/1(DCMbe)
  ulh (m)/1 -> "WGS84 Gravity Model  "/1
  Roll Torque (Nm)/1 -> Mux/2
  Thrust (N)/1 -> Sum2/2, Actuator to moment/2(Thrust (N))
  Actuator to moment/1(Thrust moment) -> Sum/1
  Xe (m)/1 -> Subsystem/4(Xe), Check if Height is 0/3(Xe (m))
  Subsystem/3(Local Airspeed (m/s)) -> Aero Forces and Moments/2(Local Airspeed (m/s))
  Subsystem/2(Mach) -> GreaterThanOrEqual/1, Aero Forces and Moments/1(Mach)
  Subsystem/4(AoA (rads)) -> Aero Forces and Moments/3(AoA (rad))
  Subsystem/5(Density (kg/m3)) -> Aero Forces and Moments/4(Density)
  Subsystem/6(Temperature (K)) -> Temperature Conversion/1, Aero Forces and Moments/5(Temperature)
  Subsystem/7(Dynamic Pressure) -> Aero Forces and Moments/6(Dynamic Pressure)
  Subsystem/8(CG location (m)) -> Aero Forces and Moments/7(Center of Mass X), Actuator to moment/1(CG Location (m)), CG Location (m)/1
  Wb (rads)/1 -> Aero Forces and Moments/8(Angular velocity (rad/s))
  Weight Force Flat earth coordinate system (N)/1 -> Sum3/1
  Sum/1 -> Sum1/2
  Sum1/1 -> Check if Height is 0/2(Moments)
  Sum2/1 -> "transform to Inertial axes "/1
  Check if Height is 0/1(Force (N)) -> Force (N)/1
  Check if Height is 0/2(Moments (Nm)) -> Moments (Nm)/1
  Body Wind Velocity (m/s)/1 -> Subsystem/2(Body Wind Velocity)
  "WGS84 Gravity Model  "/1 -> Weight Force Flat earth coordinate system (N)/1
  Constant/1 -> GreaterThanOrEqual/2
  GreaterThanOrEqual/1 -> Stop Simulation/1
  Transpose/1 -> "transform to Inertial axes "/2
  "transform to Inertial axes "/1 -> Sum3/2
  Sum3/1 -> Check if Height is 0/1(Force)
  1/1 -> Mux/1
  Mux/1 -> Sum/2
  Aero Forces and Moments/2(Aero Moments (Nm)) -> Sum1/1
  Aero Forces and Moments/1(Aero Forces (N)) -> Sum2/1

== system roll_control/Subsystem/If 0 after apogee1 ==
  In1 : Inport
  Clock1 : Clock
  Compare To Zero1 : simulink/Logic and Bit Operations/Compare To Zero  relop=<=  OutDataTypeStr=boolean
  Constant3 : Constant  Value=0.5
  Logical Operator1 : Logic  AllPortsSameDT=off  OutDataTypeStr=boolean
  Relational Operator1 : RelationalOperator  Operator=>  OutDataTypeStr=boolean  RndMeth=Simplest
  Stop Simulation1 : Stop
  wires:
  Clock1/1 -> Relational Operator1/1
  Constant3/1 -> Relational Operator1/2
  In1/1 -> Compare To Zero1/1
  Logical Operator1/1 -> Stop Simulation1/1
  Compare To Zero1/1 -> Logical Operator1/2
  Relational Operator1/1 -> Logical Operator1/1

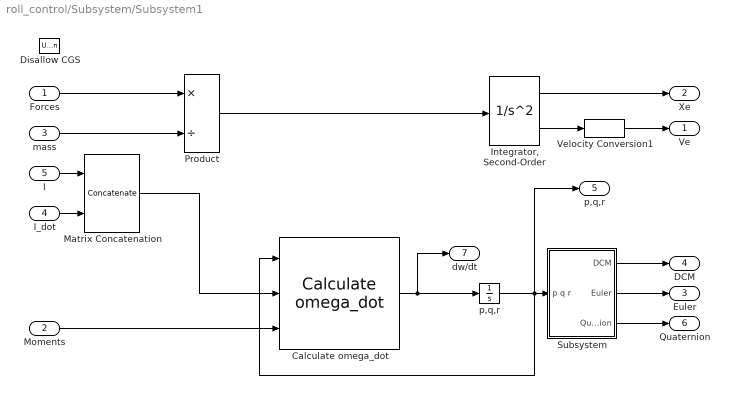
== system roll_control/Subsystem/Subsystem1 ==
  Forces : Inport  Unit=N  PortDimensions=3
  Moments : Inport  Port=2  Unit=N*m  PortDimensions=3
  mass : Inport  Port=3  Unit=kg
  I_dot : Inport  Port=4  Unit=kg*m^2/s  PortDimensions=[3 3]
  I : Inport  Port=5  Unit=kg*m^2  PortDimensions=[3 3]
  Calculate omega_dot : shared6dofsys/Calculate omega_dot  aMode=aMode
      settings: SourceProductBaseCode=AE,PW,MT,UV,VE,VP
  Disallow CGS : UnitConfiguration  UnitSystemsStr=English,SI,SI (extended)  AllowAllUnitSystems=off
  "Integrator, Second-Order" : SecondOrderIntegrator  ICX=[20; -4; 0]  LimitX=on  LowerLimitX=[-inf -inf 0]
  Matrix Concatenation : Concatenate  Mode=Multidimensional array
  Product : Product  Inputs=*/  SaturateOnIntegerOverflow=on  OutDataTypeStr=Inherit: Same as first input
  Subsystem : Subsystem
  Velocity Conversion1 : shared6dof/6DOF (Euler Angles)/Velocity Conversion1  SystemSampleTime=-1  VariantActivationTime=update diagram  Latency=0  AutoFrameSizeCalculation=off
      settings: SourceProductBaseCode=AE,PW,MT,UV,VE,VP
  "p,q,r " : Integrator  InitialCondition=[0 0 0]
  Ve : Outport  Unit=m/s  VectorParamsAs1DForOutWhenUnconnected=off
  Xe : Outport  Port=2  Unit=m  VectorParamsAs1DForOutWhenUnconnected=off
  Euler : Outport  Port=3  Unit=rad  VectorParamsAs1DForOutWhenUnconnected=off
  DCM : Outport  Port=4  Unit=1  VectorParamsAs1DForOutWhenUnconnected=off
  p,q,r : Outport  Port=5  Unit=rad/s  VectorParamsAs1DForOutWhenUnconnected=off
  Quaternion : Outport  Port=6  VectorParamsAs1DForOutWhenUnconnected=off
  dw/dt : Outport  Port=7  VectorParamsAs1DForOutWhenUnconnected=off
  wires:
  Subsystem/2(Euler) -> Euler/1
  Matrix Concatenation/1 -> Calculate omega_dot/2
  "p,q,r "/1 -> Subsystem/1(p q r), p,q,r/1, Calculate omega_dot/1
  Product/1 -> "Integrator, Second-Order"/1
  Velocity Conversion1/1 -> Ve/1
  Subsystem/1(DCM) -> DCM/1
  Calculate omega_dot/1 -> dw/dt/1, "p,q,r "/1
  I_dot/1 -> Matrix Concatenation/2
  I/1 -> Matrix Concatenation/1
  Forces/1 -> Product/1
  mass/1 -> Product/2
  Subsystem/3(Quaternion) -> Quaternion/1
  "Integrator, Second-Order"/2 -> Velocity Conversion1/1
  "Integrator, Second-Order"/1 -> Xe/1
  Moments/1 -> Calculate omega_dot/3

== system roll_control/Subsystem/Wind ==
  Rocket velocity (m/s) Ve : Inport
  DCMbe : Inport  Port=2
  Xe (m) : Inport  Port=3
  Constant : Constant  Commented=on  Value=2
  Ground : Ground  Commented=on
  Mux : Mux  Commented=on  Inputs=3
  Sel2 : Selector  InputPortWidth=3  IndexOptions=Index vector (dialog)  Indices=3  OutputSizes=1
  Subsystem3 : Subsystem
  Terminator : Terminator
  transform to body axes : shared6dof/6DOF (Euler Angles)/transform to Inertial axes   Commented=on  SystemSampleTime=-1  VariantActivationTime=update diagram  Latency=0  AutoFrameSizeCalculation=off
      settings: SourceProductBaseCode=AE,PW,MT,UV,VE,VP
  Body Wind Velocity (m/s) : Outport  VectorParamsAs1DForOutWhenUnconnected=off
  wires:
  DCMbe/1 -> Subsystem3/3(DCMbe), transform to body axes/2
  Rocket velocity (m/s) Ve/1 -> Subsystem3/1(Rocket velocity (m/s) Ve)
  Mux/1 -> transform to body axes/1
  Xe (m)/1 -> Sel2/1
  Constant/1 -> Mux/1
  Subsystem3/1(wind angular velocity (rad/s)) -> Terminator/1
  Sel2/1 -> Subsystem3/2(height (m))
  Ground/1 -> Mux/2, Mux/3
  Subsystem3/2(body axis wind velocity (m/s)) -> Body Wind Velocity (m/s)/1

== system roll_control/Subsystem3/Gain Controller ==
  w : Inport
  q : Inport  Port=2
  ref : Inport  Port=3
  Gain : Gain  Gain=-Kri  Multiplication=Matrix(K*u) (u vector)
  Integrator : Integrator
  Selector1 : Selector  InputPortWidth=3  IndexOptions=Index vector (dialog)  Indices=[2 1 3]  OutputSizes=1
  Selector2 : Selector  InputPortWidth=4  IndexOptions=Index vector (dialog)  Indices=[3 2 4]  OutputSizes=1
  Sum1 : Sum  Inputs=+-|
  Vector Concatenate4 : Concatenate  NumInputs=3
  Mb : Outport  VectorParamsAs1DForOutWhenUnconnected=off
  wires:
  Vector Concatenate4/1 -> Gain/1
  Integrator/1 -> Vector Concatenate4/3
  q/1 -> Selector2/1
  Selector1/1 -> Vector Concatenate4/1
  w/1 -> Selector1/1
  Selector2/1 -> Sum1/1, Vector Concatenate4/2
  Gain/1 -> Mb/1
  Sum1/1 -> Integrator/1
  ref/1 -> Sum1/2

== system roll_control/Subsystem3/Subsystem1 ==
  x : Inport
  y : Inport  Port=2
  z : Inport  Port=3
  Add : Sum  Inputs=-+
  Constant : Constant
  Derivative : Derivative
  Gain : Gain  Gain=2
  Magnitude Squared : Math  Operator=magnitude^2  SignedPower=on  SaturateOnIntegerOverflow=on
  Mux1 : Mux  Inputs=3
  Mux2 : Mux  Inputs=2
  Quaternion Inverse : aerolibutil/Quaternion Inverse
  Quaternion Multiplication : aerolibutil/Quaternion Multiplication
  Selector : Selector  InputPortWidth=4  IndexOptions=Index vector (dialog)  Indices=[2 3 4]  OutputSizes=1
  Sqrt : Sqrt  SaturateOnIntegerOverflow=on
  Sum of Elements : Sum  Inputs=+
  Expected angular velocity : Outport  VectorParamsAs1DForOutWhenUnconnected=off
  wires:
  Quaternion Inverse/1 -> Quaternion Multiplication/1
  x/1 -> Mux1/1
  Gain/1 -> Quaternion Multiplication/2
  Magnitude Squared/1 -> Sum of Elements/1
  Add/1 -> Sqrt/1
  Mux1/1 -> Mux2/2, Magnitude Squared/1
  Quaternion Multiplication/1 -> Selector/1
  Mux2/1 -> Quaternion Inverse/1, Derivative/1
  Constant/1 -> Add/2
  Derivative/1 -> Gain/1
  Sqrt/1 -> Mux2/1
  z/1 -> Mux1/3
  y/1 -> Mux1/2
  Sum of Elements/1 -> Add/1
  Selector/1 -> Expected angular velocity/1

== system roll_control/Subsystem3/Subsystem2 ==
  Input Acceleration : Inport  PortDimensions=[2]
  Thrust Acceleration : Inport  Port=2
  Derivative : Derivative
  Desired Quaternion : MATLAB Function  TreatAsAtomicUnit=on
  Gain : Gain  Gain=2
  Expected Quaternion : Outport  VectorParamsAs1DForOutWhenUnconnected=off
  Expected angular velocity : Outport  Port=2  VectorParamsAs1DForOutWhenUnconnected=off
  wires:
  Thrust Acceleration/1 -> Desired Quaternion/2(thrust_acceleration)
  Gain/1 -> Expected angular velocity/1
  Desired Quaternion/1(desired_quaternion) -> Expected Quaternion/1
  Derivative/1 -> Gain/1
  Desired Quaternion/2(ln_quat) -> Derivative/1
  Input Acceleration/1 -> Desired Quaternion/1(input_acceleration)

== system roll_control/Moment to Force and Actuator Model/Saturation/If 0 after apogee2 ==
  In1 : Inport
  Clock1 : Clock
  Compare To Zero1 : simulink/Logic and Bit Operations/Compare To Zero  relop=<=  OutDataTypeStr=boolean
  Constant3 : Constant  Value=2
  Logical Operator1 : Logic  AllPortsSameDT=off  OutDataTypeStr=boolean
  Relational Operator1 : RelationalOperator  Operator=>  OutDataTypeStr=boolean  RndMeth=Simplest
  Stop Simulation1 : Stop
  wires:
  Clock1/1 -> Relational Operator1/1
  Constant3/1 -> Relational Operator1/2
  In1/1 -> Compare To Zero1/1
  Logical Operator1/1 -> Stop Simulation1/1
  Compare To Zero1/1 -> Logical Operator1/2
  Relational Operator1/1 -> Logical Operator1/1

== system roll_control/Subsystem/Acceleration Calculator/Actuator to moment ==
  CG Location (m) : Inport
  Thrust (N) : Inport  Port=2
  1 : Constant  Value=[0 0]
  Constant3 : Constant  Value=.95
  Cross Product : vrlib/Utilities/Cross Product
  Gain : Gain  Gain=-1
  Mux : Mux  Inputs=2
  Sum1 : Sum  Inputs=-+|
  Thrust moment : Outport  VectorParamsAs1DForOutWhenUnconnected=off
  wires:
  Constant3/1 -> Sum1/2
  CG Location (m)/1 -> Sum1/1
  Mux/1 -> Cross Product/1
  Sum1/1 -> Gain/1
  1/1 -> Mux/1
  Thrust (N)/1 -> Cross Product/2
  Cross Product/1 -> Thrust moment/1
  Gain/1 -> Mux/2
